simulink model "p4_position"  (R2019b)
settings: Solver=VariableStepAuto  StartTime=0.0  StopTime=20  RelTol=1e-3
values from neighbouring files (symbols this model uses):
  x1_0 = 2.*rand(1,1)-1    [p1_initialization.m]    (also in p3_initialization.m; p4_initialization.m = 1)
  x2_0 = 2.*rand(1,1)-1    [p1_initialization.m]    (also in p3_initialization.m; p4_initialization.m = -1)
  x3_0 = 2.*rand(1,1)-1    [p1_initialization.m]    (also in p3_initialization.m; p4_initialization.m = 3)
  x4_0 = 2.*rand(1,1)-1    [p1_initialization.m]    (also in p3_initialization.m; p4_initialization.m = 1)
  y1_0 = 0    [p4_initialization.m]
  y2_0 = 2    [p4_initialization.m]
  y3_0 = 1    [p4_initialization.m]
  y4_0 = 1    [p4_initialization.m]
settings Model: Creator=cz  LastModifiedBy=cz

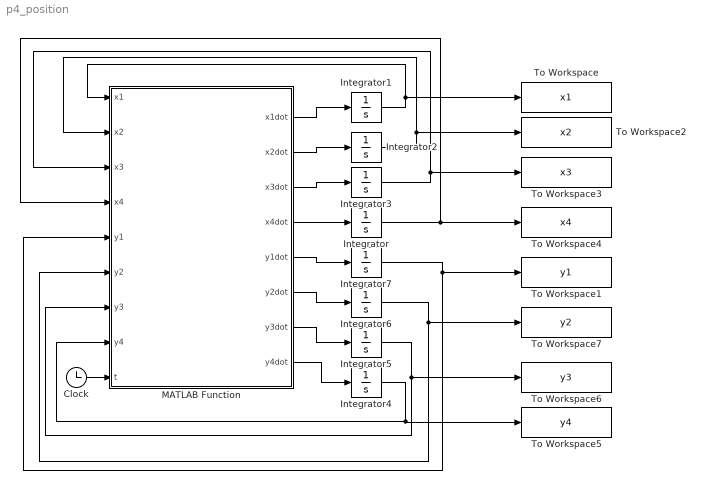
== system p4_position ==
  Clock : Clock
  Integrator : Integrator  InitialCondition=x4_0
  Integrator1 : Integrator  InitialCondition=x1_0
  Integrator2 : Integrator  InitialCondition=x2_0
  Integrator3 : Integrator  InitialCondition=x3_0
  Integrator4 : Integrator  InitialCondition=y4_0
  Integrator5 : Integrator  InitialCondition=y3_0
  Integrator6 : Integrator  InitialCondition=y2_0
  Integrator7 : Integrator  InitialCondition=y1_0
  MATLAB Function : MATLAB Function  TreatAsAtomicUnit=on
  To Workspace : ToWorkspace  VariableName=x1  SampleTime=-1
  To Workspace1 : ToWorkspace  VariableName=y1  SampleTime=-1
  To Workspace2 : ToWorkspace  VariableName=x2  SampleTime=-1
  To Workspace3 : ToWorkspace  VariableName=x3  SampleTime=-1
  To Workspace4 : ToWorkspace  VariableName=x4  SampleTime=-1
  To Workspace5 : ToWorkspace  VariableName=y4  SampleTime=-1
  To Workspace6 : ToWorkspace  VariableName=y3  SampleTime=-1
  To Workspace7 : ToWorkspace  VariableName=y2  SampleTime=-1
  wires:
  MATLAB Function/1(x1dot) -> Integrator1/1
  Integrator1/1 -> To Workspace/1, MATLAB Function/1(x1)
  MATLAB Function/2(x2dot) -> Integrator2/1
  Integrator2/1 -> MATLAB Function/2(x2), To Workspace2/1
  MATLAB Function/3(x3dot) -> Integrator3/1
  Integrator3/1 -> To Workspace3/1, MATLAB Function/3(x3)
  MATLAB Function/4(x4dot) -> Integrator/1
  Integrator/1 -> To Workspace4/1, MATLAB Function/4(x4)
  MATLAB Function/5(y1dot) -> Integrator7/1
  Clock/1 -> MATLAB Function/9(t)
  MATLAB Function/6(y2dot) -> Integrator6/1
  MATLAB Function/7(y3dot) -> Integrator5/1
  MATLAB Function/8(y4dot) -> Integrator4/1
  Integrator4/1 -> To Workspace5/1, MATLAB Function/8(y4)
  Integrator5/1 -> To Workspace6/1, MATLAB Function/7(y3)
  Integrator6/1 -> To Workspace7/1, MATLAB Function/6(y2)
  Integrator7/1 -> To Workspace1/1, MATLAB Function/5(y1)

== matlab function p4_position/MATLAB Function ==
  data: x1 input; x1dot output; x2 input; x3 input; x4 input; y1 input; y2 input; y3 input; y4 input; t input; x2dot output; x3dot output; x4dot output; y1dot output; y2dot output; y3dot output; y4dot output
function [x1dot,x2dot,x3dot,x4dot,y1dot,y2dot,y3dot,y4dot] = fcn(x1,x2,x3,x4,y1,y2,y3,y4,t)

x1dot=x4-x1;
x2dot=x1-x2+1;
x3dot=x2-x3;
x4dot=x3-x4-1;
y1dot=y4-y1+1;
y2dot=y1-y2;
y3dot=y2-y3-1;
y4dot=y3-y4;
